simulink model "ssc_battery_management_R2012b"  (R2014a)
settings: Solver=ode15s  StartTime=0.0  StopTime=2000  FixedStep=0.1  MinStep=1e-10  RelTol=1e-5
PreLoadFcn:
  | ModelPath = fileparts(get_param(bdroot,'FileName'));
  | addpath(ModelPath);
  | 
  | ssc_battery_management_R2012b_ini
values from neighbouring files (symbols this model uses):
  Kt = [0.80,1.10,1.20,1.12;]    [ssc_lead_acid_battery_50Ah_ini.m]    (also in ssc_lead_acid_battery_80Ah_ini.m)
  Kt_Temps = [25 40 60 75]    [ssc_lead_acid_battery_50Ah_ini.m]    (also in ssc_lead_acid_battery_80Ah_ini.m)
  theta_f = -40    [ssc_lead_acid_battery_50Ah_ini.m]    (also in ssc_lead_acid_battery_80Ah_ini.m)
  theta_init = 25    [ssc_lead_acid_battery_50Ah_ini.m]    (also in ssc_lead_acid_battery_80Ah_ini.m)
undefined symbols (not defined in the file or in its folder): AltData100AMaxCurrent, AltData100AVoltage, AltData80AMaxCurrent, AltData80AVoltage, DiscIntNeverNeededParam, sigbuilder_block
undefined symbols (not defined in the file): beta, center, exponent, polyTerms, WendlandNumTerms, width
libraries: fl_lib x146, LeadAcidBattery_lib x36, nesl_utility x28, simulink x1
(part 4 of 4)

== stateflow chart ssc_battery_management_R2012b/RPM Compensation/RPM Compensation- Batt Voltage ==
  settings: updateMethod=DISCRETE  sampleTime=1
  (default) -> (junction 58)
  (junction 58) -> (junction 57) [order 1] : [Integral >= 12]
  (junction 58) -> (junction 50) [order 2]
  (junction 57) -> (junction 55)
  (junction 55) -> (junction 56) [order 1] : [step1_flag == 1]
  (junction 55) -> (junction 54) [order 2] : {
      | RPM_comp += RPM_step;
      | step1_flag =1;
      | }
  (junction 56) -> (junction 53)
  (junction 53) -> (junction 54)
  (junction 54) -> (junction 43)
  (junction 43) -> (junction 44) [order 1] : [Integral >= 18]
  (junction 43) -> (junction 49) [order 2]
  (junction 44) -> (junction 52)
  (junction 50) -> (junction 45) [order 1] : [step1_flag == 0]
  (junction 50) -> (junction 40) [order 2]
  (junction 45) -> (junction 60)
  (junction 49) -> (junction 47) [order 1] : [step2_flag == 1]
  (junction 49) -> (junction 48) [order 2]
  (junction 47) -> (junction 38)
  (junction 40) -> (junction 46) [order 1] : [Integral < 2]
  (junction 52) -> (junction 35) [order 1] : [step2_flag == 1]
  (junction 38) -> (junction 37) [order 1] : [Integral < 17]
  (junction 40) -> (junction 42) [order 2]
  (junction 46) -> (junction 41) : {
      | RPM_comp += RPM_step;
      | step1_flag = 0;
      | }
  (junction 52) -> (junction 36) [order 2] : {
      | RPM_comp += RPM_step;
      | step2_flag = 1;
      | }
  (junction 35) -> (junction 59)
  (junction 38) -> (junction 51) [order 2]
  (junction 37) -> (junction 39) : {
      | RPM_comp -= RPM_step;
      | step2_flag = 0;
      | }
  (junction 41) -> (junction 42)
  (junction 60) -> (junction 41)
  (junction 48) -> (junction 60)
  (junction 51) -> (junction 48)
  (junction 39) -> (junction 51)
  (junction 36) -> (junction 39)
  (junction 59) -> (junction 36)
  data: RPM_comp output double; step1_flag output boolean; step2_flag output boolean; Integral input; RPM_step input
